simulink model "Simulation_der_Modelle"  (R2016a)
settings: Solver=FixedStepAuto  StartTime=0.0  StopTime=200.0  FixedStep=T_s  RelTol=1e-3
values from neighbouring files (symbols this model uses):
  AC1 = (1/J)*(0.5*rho*pi*R^4*v_c*CM_dlambda)    [Regerlung_einer_WEA.m]
  AC2 = [(-d_s/J_r)+(0.5*rho*pi*R^4*v_c*CM_dlambda)/J_r,-k_s/J_r,(d_s*n_g_inv)/J_r,(k_s*n_g_inv)/J_r ... (first row only)    [Regerlung_einer_WEA.m]
  AC3 = [((1/J_r)*((0.5*rho*pi*R^4*v_c*CM_dlambda)-d_s)),(-1/J_r)*k_s,(1/J_r)*d_s*n_g_inv,(1/J_r)*k_s*n_g_inv,0,0 ... (first row only)    [Regerlung_einer_WEA.m]
  AC4 = [(-d_s/J_r)+(0.5*rho*pi*R^4*v_c*CM_dlambda)/J_r,-k_s/J_r,(d_s*n_g_inv)/J_r,(k_s*n_g_inv)/J_r,0,0,0,0 ... (first row only)    [Regerlung_einer_WEA.m]
  AD1 = expm(AC1*T_s)    [Regerlung_einer_WEA.m]
  AD2 = expm(AC2*T_s)    [Regerlung_einer_WEA.m]
  AD3 = expm(AC3*T_s)    [Regerlung_einer_WEA.m]
  AD4 = expm(AC4*T_s)    [Regerlung_einer_WEA.m]
  BC1 = [(1/J)*(0.5*rho*R^3*v_c^2*CM_dtheta),(-1/J)*n_g,(1/J)*((-rho*pi*R^4*w_r_c)*CM_dlambda+rho*pi*R^3*v_c*CM)]    [Regerlung_einer_WEA.m]
  BC2 = [(0.5*rho*pi*R^3*v_c^2*CM_dtheta)/J_r,0,(-0.5*pi*rho*R^4*w_r_c*CM_dlambda)/J_r+(rho*pi*R^3*v_c*CM)/J_r ... (first row only)    [Regerlung_einer_WEA.m]
  BC3 = [(1/J_r)*0.5*rho*pi*R^3*v_c^2*CM_dtheta,0,(1/J_r)*((-0.5*rho*pi*R^4*w_r_c)*CM_dlambda+rho*pi*R^3*v_c*CM) ... (first row only)    [Regerlung_einer_WEA.m]
  BC4 = [(0.5*rho*pi*R^3*v_c^2*CM_dtheta)/J_r,0,(-0.5*pi*rho*R^4*w_r_c*CM_dlambda)/J_r+(rho*pi*R^3*v_c*CM)/J_r ... (first row only)    [Regerlung_einer_WEA.m]
  BD1 = inv(AC1)*(expm(AC1*T_s)-I1)*BC1    [Regerlung_einer_WEA.m]
  BD2 = inv(AC2)*(expm(AC2*T_s)-I2)*BC2    [Regerlung_einer_WEA.m]
  BD3 = inv(AC3)*(expm(AC3*T_s)-I3)*BC3    [Regerlung_einer_WEA.m]
  BD4 = inv(AC4)*(expm(AC4*T_s)-I4)*BC4    [Regerlung_einer_WEA.m]
  C1 = zeors(s1*Nu,s1)    [OptimierungMitConstrains.m]    (also in Regerlung_einer_WEA.m = 1)
  C2 = zeors(s1*Nu,s1*Nu)    [OptimierungMitConstrains.m]    (also in Regerlung_einer_WEA.m = [1,0,0,0])
  C3 = [1,0,0,0,0,0 ... (first row only)    [Regerlung_einer_WEA.m]
  C4 = [1,0,0,0,0,0,0,0 ... (first row only)    [Regerlung_einer_WEA.m]
  D1 = zeros(1,3)    [Regerlung_einer_WEA.m]
  D2 = zeros(1,3)    [Regerlung_einer_WEA.m]
  D3 = zeros(3,3)    [Regerlung_einer_WEA.m]
  D4 = zeros(5,3)    [Regerlung_einer_WEA.m]
  T_s = 0.05    [Regerlung_einer_WEA.m]
settings Model: Creator=pasca  LastModifiedBy=pasca

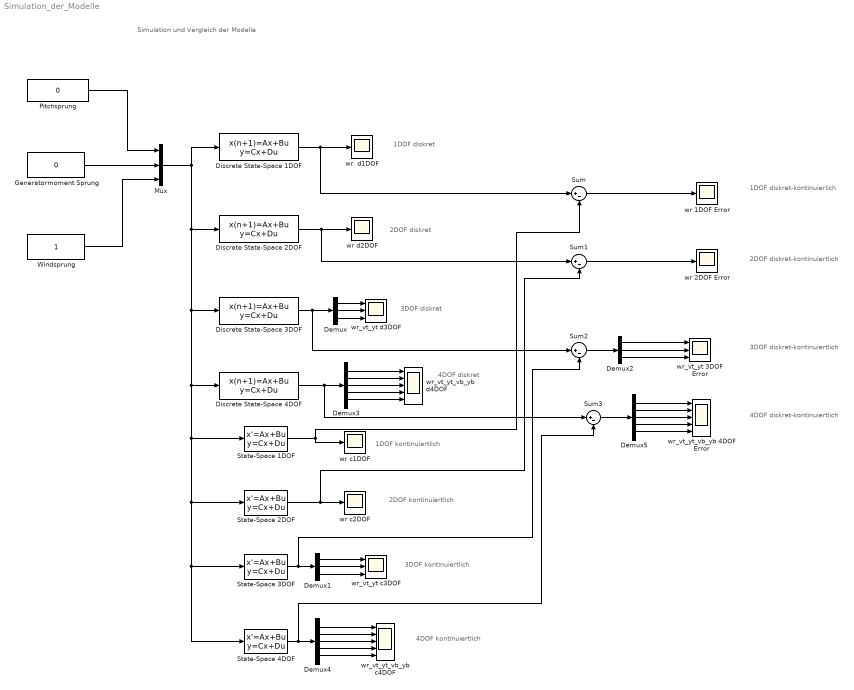
== system Simulation_der_Modelle ==
  note: Simulation und Vergleich der Modelle
  note: 1DOF diskret-kontinuierlich
  note: 1DOF diskret
  note: 2DOF diskret
  note: 3DOF diskret
  note: 4DOF diskret
  note: 1DOF kontinuiertlich
  note: 2DOF kontinuiertlich
  note: 3DOF kontinuiertlich
  note: 4DOF kontinuiertlich
  note: 2DOF diskret-kontinuiertlich
  note: 3DOF diskret-kontinuiertlich
  note: 4DOF diskret-kontinuiertlich
  " wr 1DOF Error" : Scope
  Demux : Demux  Outputs=3
  Demux1 : Demux  Outputs=3
  Demux2 : Demux  Outputs=3
  Demux3 : Demux  Outputs=5
  Demux4 : Demux  Outputs=5
  Demux5 : Demux  Outputs=5
  Discrete State-Space 1DOF : DiscreteStateSpace  A=AD1  B=BD1  C=C1  D=D1  SampleTime=T_s
  Discrete State-Space 2DOF : DiscreteStateSpace  A=AD2  B=BD2  C=C2  D=D2  SampleTime=T_s
  Discrete State-Space 3DOF : DiscreteStateSpace  A=AD3  B=BD3  C=C3  D=D3  SampleTime=T_s
  Discrete State-Space 4DOF : DiscreteStateSpace  A=AD4  B=BD4  C=C4  D=D4  SampleTime=T_s
  Generatormoment Sprung : Constant  Value=0
  Mux : Mux  Inputs=3
  Pitchsprung : Constant  Value=0
  "State-Space 1DOF " : StateSpace  A=AC1  B=BC1  C=C1  D=D1  X0=0
  State-Space 2DOF : StateSpace  A=AC2  B=BC2  C=C2  D=D2  X0=0
  "State-Space 3DOF " : StateSpace  A=AC3  B=BC3  C=C3  D=D3  X0=0
  State-Space 4DOF : StateSpace  A=AC4  B=BC4  C=C4  D=D4  X0=0
  Sum{,1..3} (4 alike) : Sum  Inputs=|+-
  Windsprung : Constant
  wr  d1DOF : Scope
  wr 2DOF Error : Scope
  "wr c1DOF " : Scope
  wr c2DOF : Scope
  wr d2DOF : Scope
  wr_vt_yt 3DOF Error : Scope  NumInputPorts=3
  wr_vt_yt c3DOF : Scope  NumInputPorts=3
  "wr_vt_yt d3DOF " : Scope  NumInputPorts=3
  wr_vt_yt_vb_yb 4DOF Error : Scope  NumInputPorts=5
  wr_vt_yt_vb_yb c4DOF : Scope  NumInputPorts=5
  "wr_vt_yt_vb_yb d4DOF " : Scope  NumInputPorts=5
  wires:
  Pitchsprung/1 -> Mux/1
  Generatormoment Sprung/1 -> Mux/2
  Mux/1 -> Discrete State-Space 1DOF/1, Discrete State-Space 4DOF/1, State-Space 4DOF/1, "State-Space 3DOF "/1, State-Space 2DOF/1, "State-Space 1DOF "/1, Discrete State-Space 3DOF/1, Discrete State-Space 2DOF/1
  Discrete State-Space 2DOF/1 -> Sum1/1, wr d2DOF/1
  Windsprung/1 -> Mux/3
  Demux/1 -> "wr_vt_yt d3DOF "/1
  Discrete State-Space 3DOF/1 -> Sum2/1, Demux/1
  Demux/2 -> "wr_vt_yt d3DOF "/2
  Demux/3 -> "wr_vt_yt d3DOF "/3
  State-Space 2DOF/1 -> Sum1/2, wr c2DOF/1
  "State-Space 1DOF "/1 -> "wr c1DOF "/1, Sum/2
  "State-Space 3DOF "/1 -> Sum2/2, Demux1/1
  Demux1/1 -> wr_vt_yt c3DOF/1
  Demux1/2 -> wr_vt_yt c3DOF/2
  Demux1/3 -> wr_vt_yt c3DOF/3
  Discrete State-Space 1DOF/1 -> Sum/1, wr  d1DOF/1
  Sum/1 -> " wr 1DOF Error"/1
  Sum1/1 -> wr 2DOF Error/1
  Sum2/1 -> Demux2/1
  Demux2/1 -> wr_vt_yt 3DOF Error/1
  Demux2/2 -> wr_vt_yt 3DOF Error/2
  Demux2/3 -> wr_vt_yt 3DOF Error/3
  Demux3/1 -> "wr_vt_yt_vb_yb d4DOF "/1
  Demux3/2 -> "wr_vt_yt_vb_yb d4DOF "/2
  Demux3/3 -> "wr_vt_yt_vb_yb d4DOF "/3
  Discrete State-Space 4DOF/1 -> Sum3/1, Demux3/1
  Demux3/5 -> "wr_vt_yt_vb_yb d4DOF "/5
  Demux3/4 -> "wr_vt_yt_vb_yb d4DOF "/4
  Demux4/1 -> wr_vt_yt_vb_yb c4DOF/1
  Demux4/2 -> wr_vt_yt_vb_yb c4DOF/2
  Demux4/3 -> wr_vt_yt_vb_yb c4DOF/3
  Demux4/5 -> wr_vt_yt_vb_yb c4DOF/5
  Demux4/4 -> wr_vt_yt_vb_yb c4DOF/4
  Demux5/1 -> wr_vt_yt_vb_yb 4DOF Error/1
  Demux5/2 -> wr_vt_yt_vb_yb 4DOF Error/2
  Demux5/3 -> wr_vt_yt_vb_yb 4DOF Error/3
  Demux5/5 -> wr_vt_yt_vb_yb 4DOF Error/5
  Demux5/4 -> wr_vt_yt_vb_yb 4DOF Error/4
  State-Space 4DOF/1 -> Sum3/2, Demux4/1
  Sum3/1 -> Demux5/1
